simulink model "test"  (R2013a)
settings: Solver=FixedStepDiscrete  StartTime=0.0  StopTime=20.0  FixedStep=0.05  RelTol=1e-3
libraries: lib_darwinop x1, utility x1
settings Model: SimulationMode=accelerator  Creator=florent  LastModifiedBy=florent

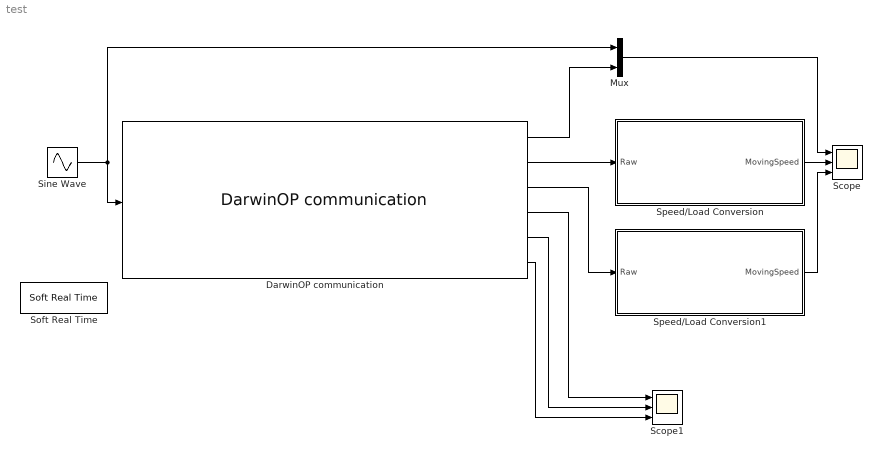
== system test ==
  DarwinOP communication : lib_darwinop/DarwinOP communication  IP=192.168.123.1  Port=1234  Protocol=tcp  Timeout=1.0  Frame=[ 2 1 36 6 3 1 30 2 0 0 2 200 44 6]  ReadIndex=[ 1 2;3 2;5 2;7 2;9 2;11 2]  WriteIndex=[ 9 2]
  Mux : Mux  Inputs=2
  Scope : Scope  NumInputPorts=3
      settings: YMin=1000~-100~-700  YMax=3000~475~200
  Scope1 : Scope  NumInputPorts=3
      settings: YMin=507~505~622.5  YMax=519~535~655
  Sine Wave : Sin  Amplitude=1000  Bias=2000  SampleTime=0.05
  Soft Real Time : utility/Soft Real Time  x=1
  Speed/Load Conversion : MATLAB Function  TreatAsAtomicUnit=on
  Speed/Load Conversion1 : MATLAB Function  TreatAsAtomicUnit=on
  wires:
  Sine Wave/1 -> DarwinOP communication/1, Mux/1
  DarwinOP communication/1 -> Mux/2
  DarwinOP communication/3 -> Speed/Load Conversion1/1(Raw)
  DarwinOP communication/2 -> Speed/Load Conversion/1(Raw)
  Speed/Load Conversion/1(MovingSpeed) -> Scope/2
  Speed/Load Conversion1/1(MovingSpeed) -> Scope/3
  Mux/1 -> Scope/1
  DarwinOP communication/4 -> Scope1/1
  DarwinOP communication/5 -> Scope1/2
  DarwinOP communication/6 -> Scope1/3

== matlab function test/Speed//Load Conversion1 ==
  data: Raw input; MovingSpeed output
function MovingSpeed = fcn(Raw)
%#codegen

Raw16 = uint16(Raw);
if bitand(Raw16,1024) ~= 0
    MovingSpeed = -double(bitand(Raw16,1023));
else
    MovingSpeed = double(bitand(Raw16,1023));
end

== matlab function test/Speed//Load Conversion ==
  data: Raw input; MovingSpeed output
function MovingSpeed = fcn(Raw)
%#codegen

Raw16 = uint16(Raw);
if bitand(Raw16,1024) ~= 0
    MovingSpeed = -double(bitand(Raw16,1023));
else
    MovingSpeed = double(bitand(Raw16,1023));
end
